simulink library "starslibAxisTransformations"  (R2024b)
settings: Solver=ode45  StartTime=0.0  StopTime=10.0  RelTol=1e-3  EnableMultiTasking=on
libraries: starslibMathOperations x25, $bdroot x18
(part 2 of 2)

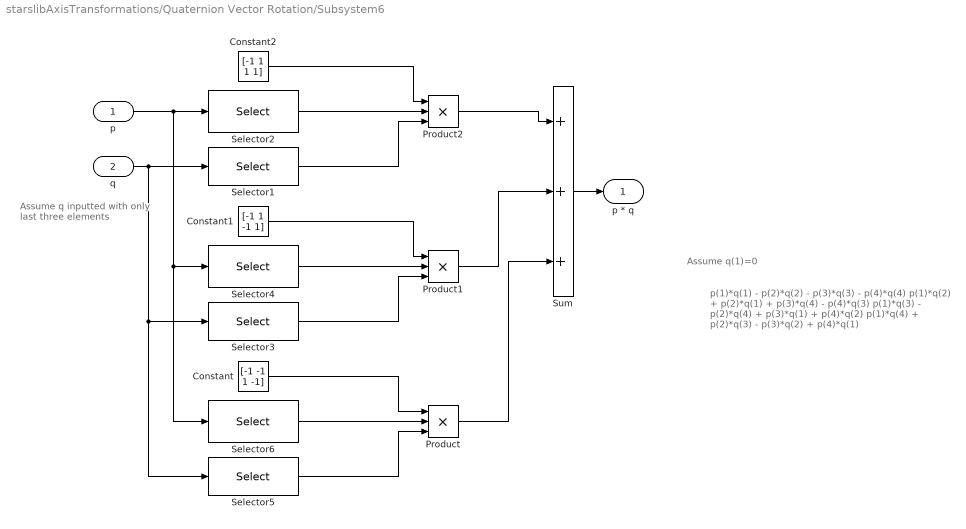
== system starslibAxisTransformations/Quaternion Vector Rotation/Subsystem6 ==
  note: p(1)*q(1) - p(2)*q(2) - p(3)*q(3) - p(4)*q(4)
      |
      | p(1)*q(2) + p(2)*q(1) + p(3)*q(4) - p(4)*q(3)
      |
      | p(1)*q(3) - p(2)*q(4) + p(3)*q(1) + p(4)*q(2)
      |
      | p(1)*q(4) + p(2)*q(3) - p(3)*q(2) + p(4)*q(1)
  note: Assume q(1)=0
  note: Assume q
      | inputted with only
      | last three elements
  p : Inport
  q : Inport  Port=2
  Constant : Constant  Value=[-1 -1 1 -1]
  Constant1 : Constant  Value=[-1 1 -1 1]
  Constant2 : Constant  Value=[-1 1 1 1]
  Product : Product  Inputs=3  RndMeth=Zero
  Product1 : Product  Inputs=3  RndMeth=Zero
  Product2 : Product  Inputs=3  RndMeth=Zero
  Selector1 : Selector  InputPortWidth=3  IndexOptions=Index vector (dialog)  Indices=[1 1 2 3]  OutputSizes=1
  Selector2 : Selector  InputPortWidth=4  IndexOptions=Index vector (dialog)  Indices=[2 1 1 1]  OutputSizes=1
  Selector3 : Selector  InputPortWidth=3  IndexOptions=Index vector (dialog)  Indices=[2 3 3 2]  OutputSizes=1
  Selector4 : Selector  InputPortWidth=4  IndexOptions=Index vector (dialog)  Indices=[3 3 2 2]  OutputSizes=1
  Selector5 : Selector  InputPortWidth=3  IndexOptions=Index vector (dialog)  Indices=[3 2 1 1]  OutputSizes=1
  Selector6 : Selector  InputPortWidth=4  IndexOptions=Index vector (dialog)  Indices=[4 4 4 3]  OutputSizes=1
  Sum : Sum  Inputs=+++
  p * q : Outport
  wires:
  Constant1/1 -> Product1/1
  Constant2/1 -> Product2/1
  Constant/1 -> Product/1
  Selector4/1 -> Product1/2
  Selector6/1 -> Product/2
  Selector1/1 -> Product2/3
  Selector3/1 -> Product1/3
  Selector5/1 -> Product/3
  Product2/1 -> Sum/1
  Product1/1 -> Sum/2
  Product/1 -> Sum/3
  p/1 -> Selector2/1, Selector4/1, Selector6/1
  q/1 -> Selector1/1, Selector3/1, Selector5/1
  Sum/1 -> p * q/1
  Selector2/1 -> Product2/2

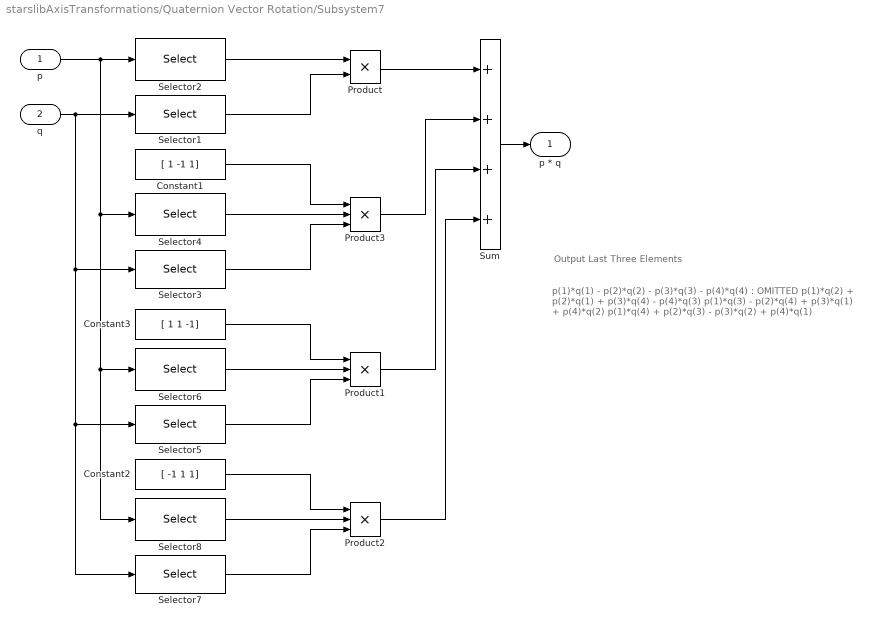
== system starslibAxisTransformations/Quaternion Vector Rotation/Subsystem7 ==
  note: Output Last Three Elements
  note: p(1)*q(1) - p(2)*q(2) - p(3)*q(3) - p(4)*q(4) :  OMITTED
      |
      | p(1)*q(2) + p(2)*q(1) + p(3)*q(4) - p(4)*q(3)
      |
      | p(1)*q(3) - p(2)*q(4) + p(3)*q(1) + p(4)*q(2)
      |
      | p(1)*q(4) + p(2)*q(3) - p(3)*q(2) + p(4)*q(1)
  p : Inport
  q : Inport  Port=2
  Constant1 : Constant  Value=[ 1 -1 1]
  Constant2 : Constant  Value=[ -1 1 1]
  Constant3 : Constant  Value=[ 1 1 -1]
  Product : Product  RndMeth=Zero
  Product1 : Product  Inputs=3  RndMeth=Zero
  Product2 : Product  Inputs=3  RndMeth=Zero
  Product3 : Product  Inputs=3  RndMeth=Zero
  Selector1 : Selector  InputPortWidth=4  IndexOptions=Index vector (dialog)  Indices=[ 2 3 4]  OutputSizes=1
  Selector2 : Selector  InputPortWidth=4  IndexOptions=Index vector (dialog)  Indices=[ 1 1 1]  OutputSizes=1
  Selector3 : Selector  InputPortWidth=4  IndexOptions=Index vector (dialog)  Indices=[ 1 4 3]  OutputSizes=1
  Selector4 : Selector  InputPortWidth=4  IndexOptions=Index vector (dialog)  Indices=[ 2 2 2]  OutputSizes=1
  Selector5 : Selector  InputPortWidth=4  IndexOptions=Index vector (dialog)  Indices=[ 4 1 2]  OutputSizes=1
  Selector6 : Selector  InputPortWidth=4  IndexOptions=Index vector (dialog)  Indices=[ 3 3 3]  OutputSizes=1
  Selector7 : Selector  InputPortWidth=4  IndexOptions=Index vector (dialog)  Indices=[ 3 2 1]  OutputSizes=1
  Selector8 : Selector  InputPortWidth=4  IndexOptions=Index vector (dialog)  Indices=[4 4 4]  OutputSizes=1
  Sum : Sum  Inputs=++++
  p * q : Outport
  wires:
  Selector5/1 -> Product1/3
  Selector6/1 -> Product1/2
  Constant3/1 -> Product1/1
  Selector7/1 -> Product2/3
  Selector8/1 -> Product2/2
  Constant2/1 -> Product2/1
  Selector3/1 -> Product3/3
  Selector4/1 -> Product3/2
  Constant1/1 -> Product3/1
  Selector1/1 -> Product/2
  Selector2/1 -> Product/1
  Sum/1 -> p * q/1
  q/1 -> Selector7/1, Selector5/1, Selector3/1, Selector1/1
  p/1 -> Selector8/1, Selector6/1, Selector4/1, Selector2/1
  Product2/1 -> Sum/4
  Product1/1 -> Sum/3
  Product3/1 -> Sum/2
  Product/1 -> Sum/1

== system starslibAxisTransformations/nQuaternion Decomposition/Divide by Zero Protection ==
  note: Replace magnitudes equal to 0 by 1
  M : Inport
  Constant : Constant
  Switch : Switch  Criteria=u2 ~= 0  ZeroCross=off  SaturateOnIntegerOverflow=off  InputSameDT=off
  M* : Outport
  wires:
  M/1 -> Switch/1, Switch/2
  Constant/1 -> Switch/3
  Switch/1 -> M*/1

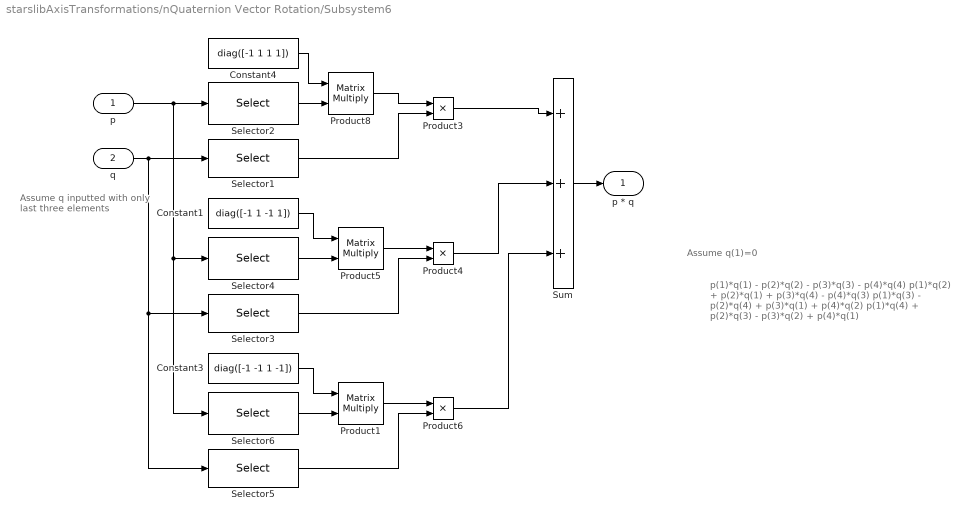
== system starslibAxisTransformations/nQuaternion Vector Rotation/Subsystem6 ==
  note: Assume q
      | inputted with only
      | last three elements
  note: Assume q(1)=0
  note: p(1)*q(1) - p(2)*q(2) - p(3)*q(3) - p(4)*q(4)
      |
      | p(1)*q(2) + p(2)*q(1) + p(3)*q(4) - p(4)*q(3)
      |
      | p(1)*q(3) - p(2)*q(4) + p(3)*q(1) + p(4)*q(2)
      |
      | p(1)*q(4) + p(2)*q(3) - p(3)*q(2) + p(4)*q(1)
  p : Inport  PortDimensions=[4,nQuat]
  q : Inport  Port=2  PortDimensions=[3,nQuat]
  Constant1 : Constant  Value=diag([-1 1 -1 1])  VectorParams1D=off
  Constant3 : Constant  Value=diag([-1 -1 1 -1])  VectorParams1D=off
  Constant4 : Constant  Value=diag([-1 1 1 1])  VectorParams1D=off
  Product1 : Product  Multiplication=Matrix(*)  RndMeth=Zero
  Product3 : Product  RndMeth=Zero
  Product4 : Product  RndMeth=Zero
  Product5 : Product  Multiplication=Matrix(*)  RndMeth=Zero
  Product6 : Product  RndMeth=Zero
  Product8 : Product  Multiplication=Matrix(*)  RndMeth=Zero
  Selector1 : Selector  NumberOfDimensions=2  InputPortWidth=3  IndexOptions=Index vector (dialog),Select all  Indices=[1 1 2 3],1  OutputSizes=1,1
  Selector2 : Selector  NumberOfDimensions=2  InputPortWidth=3  IndexOptions=Index vector (dialog),Select all  Indices=[2 1 1 1],1  OutputSizes=1,1
  Selector3 : Selector  NumberOfDimensions=2  InputPortWidth=3  IndexOptions=Index vector (dialog),Select all  Indices=[2 3 3 2],1  OutputSizes=1,1
  Selector4 : Selector  NumberOfDimensions=2  InputPortWidth=3  IndexOptions=Index vector (dialog),Select all  Indices=[3 3 2 2],1  OutputSizes=1,1
  Selector5 : Selector  NumberOfDimensions=2  InputPortWidth=3  IndexOptions=Index vector (dialog),Select all  Indices=[3 2 1 1],1  OutputSizes=1,1
  Selector6 : Selector  NumberOfDimensions=2  InputPortWidth=3  IndexOptions=Index vector (dialog),Select all  Indices=[4 4 4 3],1  OutputSizes=1,1
  Sum : Sum  Inputs=+++
  p * q : Outport  PortDimensions=[4,nQuat]
  wires:
  Constant4/1 -> Product8/1
  Product8/1 -> Product3/1
  Selector2/1 -> Product8/2
  Sum/1 -> p * q/1
  q/1 -> Selector5/1, Selector3/1, Selector1/1
  p/1 -> Selector6/1, Selector4/1, Selector2/1
  Product6/1 -> Sum/3
  Product4/1 -> Sum/2
  Product3/1 -> Sum/1
  Selector5/1 -> Product6/2
  Product1/1 -> Product6/1
  Selector3/1 -> Product4/2
  Product5/1 -> Product4/1
  Selector1/1 -> Product3/2
  Constant3/1 -> Product1/1
  Selector6/1 -> Product1/2
  Constant1/1 -> Product5/1
  Selector4/1 -> Product5/2

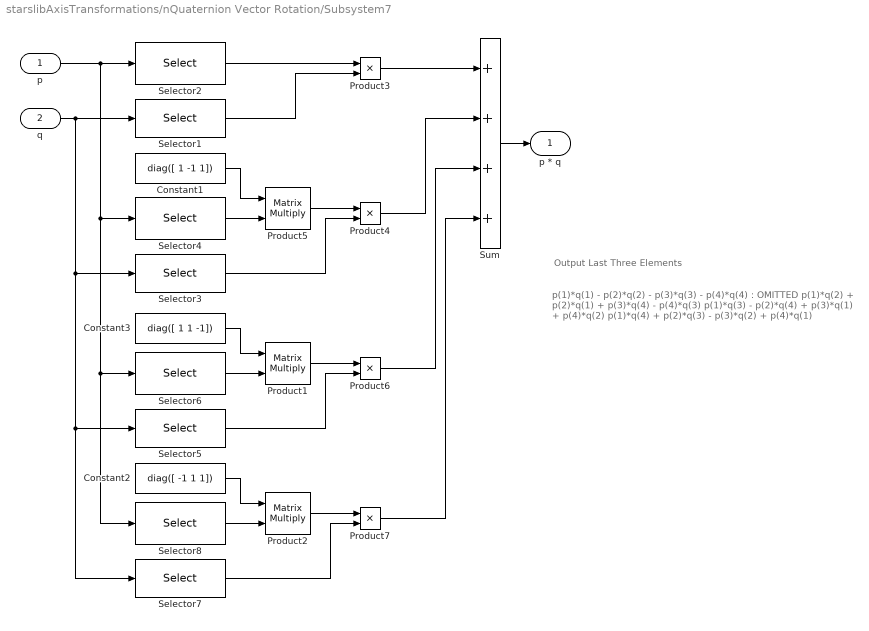
== system starslibAxisTransformations/nQuaternion Vector Rotation/Subsystem7 ==
  note: Output Last Three Elements
  note: p(1)*q(1) - p(2)*q(2) - p(3)*q(3) - p(4)*q(4) :  OMITTED
      |
      | p(1)*q(2) + p(2)*q(1) + p(3)*q(4) - p(4)*q(3)
      |
      | p(1)*q(3) - p(2)*q(4) + p(3)*q(1) + p(4)*q(2)
      |
      | p(1)*q(4) + p(2)*q(3) - p(3)*q(2) + p(4)*q(1)
  p : Inport  PortDimensions=[4,nQuat]
  q : Inport  Port=2  PortDimensions=[4,nQuat]
  Constant1 : Constant  Value=diag([ 1 -1 1])  VectorParams1D=off
  Constant2 : Constant  Value=diag([ -1 1 1])  VectorParams1D=off
  Constant3 : Constant  Value=diag([ 1 1 -1])  VectorParams1D=off
  Product1 : Product  Multiplication=Matrix(*)  RndMeth=Zero
  Product2 : Product  Multiplication=Matrix(*)  RndMeth=Zero
  Product{3..4,6..7} (4 alike) : Product  RndMeth=Zero
  Product5 : Product  Multiplication=Matrix(*)  RndMeth=Zero
  Selector1 : Selector  NumberOfDimensions=2  InputPortWidth=3  IndexOptions=Index vector (dialog),Select all  Indices=[ 2 3 4],1  OutputSizes=1,1
  Selector2 : Selector  NumberOfDimensions=2  InputPortWidth=3  IndexOptions=Index vector (dialog),Select all  Indices=[ 1 1 1],1  OutputSizes=1,1
  Selector3 : Selector  NumberOfDimensions=2  InputPortWidth=3  IndexOptions=Index vector (dialog),Select all  Indices=[ 1 4 3],1  OutputSizes=1,1
  Selector4 : Selector  NumberOfDimensions=2  InputPortWidth=3  IndexOptions=Index vector (dialog),Select all  Indices=[ 2 2 2],1  OutputSizes=1,1
  Selector5 : Selector  NumberOfDimensions=2  InputPortWidth=3  IndexOptions=Index vector (dialog),Select all  Indices=[ 4 1 2],1  OutputSizes=1,1
  Selector6 : Selector  NumberOfDimensions=2  InputPortWidth=3  IndexOptions=Index vector (dialog),Select all  Indices=[ 3 3 3],1  OutputSizes=1,1
  Selector7 : Selector  NumberOfDimensions=2  InputPortWidth=3  IndexOptions=Index vector (dialog),Select all  Indices=[ 3 2 1],1  OutputSizes=1,1
  Selector8 : Selector  NumberOfDimensions=2  InputPortWidth=3  IndexOptions=Index vector (dialog),Select all  Indices=[4 4 4],1  OutputSizes=1,1
  Sum : Sum  Inputs=++++
  p * q : Outport  PortDimensions=[3,nQuat]
  wires:
  Sum/1 -> p * q/1
  q/1 -> Selector7/1, Selector5/1, Selector3/1, Selector1/1
  p/1 -> Selector8/1, Selector6/1, Selector4/1, Selector2/1
  Product7/1 -> Sum/4
  Product6/1 -> Sum/3
  Product4/1 -> Sum/2
  Product3/1 -> Sum/1
  Selector7/1 -> Product7/2
  Product2/1 -> Product7/1
  Selector5/1 -> Product6/2
  Product1/1 -> Product6/1
  Selector3/1 -> Product4/2
  Product5/1 -> Product4/1
  Selector1/1 -> Product3/2
  Selector2/1 -> Product3/1
  Constant2/1 -> Product2/1
  Selector8/1 -> Product2/2
  Constant3/1 -> Product1/1
  Selector6/1 -> Product1/2
  Constant1/1 -> Product5/1
  Selector4/1 -> Product5/2

== system starslibAxisTransformations/slkQuaternion Vector Rotation/Subsystem6 ==
  note: Assume q
      | inputted with only
      | last three elements
  note: Assume q(1)=0
  note: p(1)*q(1) - p(2)*q(2) - p(3)*q(3) - p(4)*q(4)
      |
      | p(1)*q(2) + p(2)*q(1) + p(3)*q(4) - p(4)*q(3)
      |
      | p(1)*q(3) - p(2)*q(4) + p(3)*q(1) + p(4)*q(2)
      |
      | p(1)*q(4) + p(2)*q(3) - p(3)*q(2) + p(4)*q(1)
  p : Inport
  q : Inport  Port=2
  Constant : Constant  Value=[-1 -1 1 -1]
  Constant1 : Constant  Value=[-1 1 -1 1]
  Constant2 : Constant  Value=[-1 1 1 1]
  Product : Product  Inputs=3  RndMeth=Zero
  Product1 : Product  Inputs=3  RndMeth=Zero
  Product2 : Product  Inputs=3  RndMeth=Zero
  Selector1 : Selector  InputPortWidth=3  IndexOptions=Index vector (dialog)  Indices=[1 1 2 3]  OutputSizes=1
  Selector2 : Selector  InputPortWidth=4  IndexOptions=Index vector (dialog)  Indices=[2 1 1 1]  OutputSizes=1
  Selector3 : Selector  InputPortWidth=3  IndexOptions=Index vector (dialog)  Indices=[2 3 3 2]  OutputSizes=1
  Selector4 : Selector  InputPortWidth=4  IndexOptions=Index vector (dialog)  Indices=[3 3 2 2]  OutputSizes=1
  Selector5 : Selector  InputPortWidth=3  IndexOptions=Index vector (dialog)  Indices=[3 2 1 1]  OutputSizes=1
  Selector6 : Selector  InputPortWidth=4  IndexOptions=Index vector (dialog)  Indices=[4 4 4 3]  OutputSizes=1
  Sum : Sum  Inputs=+++
  p * q : Outport
  wires:
  Selector2/1 -> Product2/2
  Sum/1 -> p * q/1
  q/1 -> Selector5/1, Selector3/1, Selector1/1
  p/1 -> Selector6/1, Selector4/1, Selector2/1
  Product/1 -> Sum/3
  Product1/1 -> Sum/2
  Product2/1 -> Sum/1
  Selector5/1 -> Product/3
  Selector3/1 -> Product1/3
  Selector1/1 -> Product2/3
  Selector6/1 -> Product/2
  Selector4/1 -> Product1/2
  Constant/1 -> Product/1
  Constant2/1 -> Product2/1
  Constant1/1 -> Product1/1

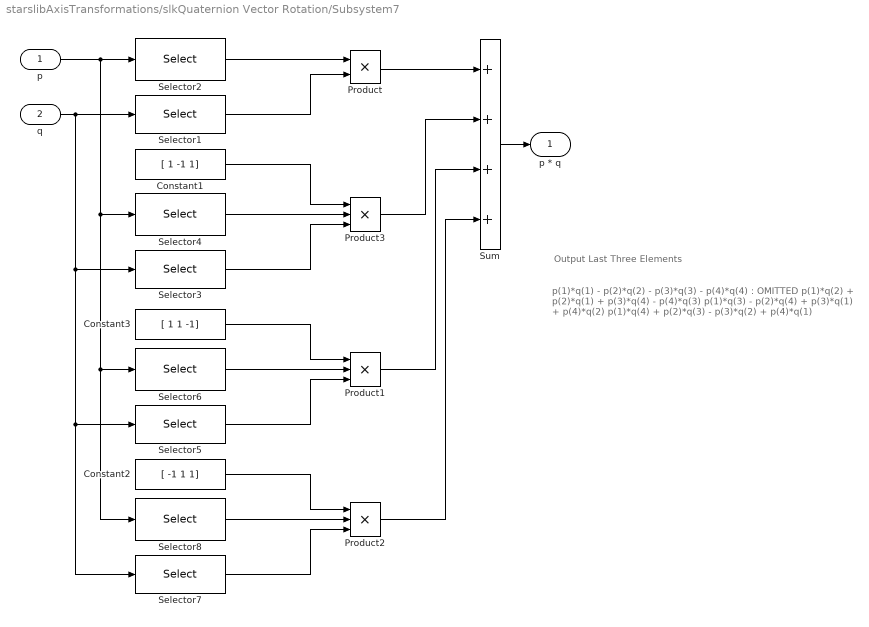
== system starslibAxisTransformations/slkQuaternion Vector Rotation/Subsystem7 ==
  note: p(1)*q(1) - p(2)*q(2) - p(3)*q(3) - p(4)*q(4) :  OMITTED
      |
      | p(1)*q(2) + p(2)*q(1) + p(3)*q(4) - p(4)*q(3)
      |
      | p(1)*q(3) - p(2)*q(4) + p(3)*q(1) + p(4)*q(2)
      |
      | p(1)*q(4) + p(2)*q(3) - p(3)*q(2) + p(4)*q(1)
  note: Output Last Three Elements
  p : Inport
  q : Inport  Port=2
  Constant1 : Constant  Value=[ 1 -1 1]
  Constant2 : Constant  Value=[ -1 1 1]
  Constant3 : Constant  Value=[ 1 1 -1]
  Product : Product  RndMeth=Zero
  Product1 : Product  Inputs=3  RndMeth=Zero
  Product2 : Product  Inputs=3  RndMeth=Zero
  Product3 : Product  Inputs=3  RndMeth=Zero
  Selector1 : Selector  InputPortWidth=4  IndexOptions=Index vector (dialog)  Indices=[ 2 3 4]  OutputSizes=1
  Selector2 : Selector  InputPortWidth=4  IndexOptions=Index vector (dialog)  Indices=[ 1 1 1]  OutputSizes=1
  Selector3 : Selector  InputPortWidth=4  IndexOptions=Index vector (dialog)  Indices=[ 1 4 3]  OutputSizes=1
  Selector4 : Selector  InputPortWidth=4  IndexOptions=Index vector (dialog)  Indices=[ 2 2 2]  OutputSizes=1
  Selector5 : Selector  InputPortWidth=4  IndexOptions=Index vector (dialog)  Indices=[ 4 1 2]  OutputSizes=1
  Selector6 : Selector  InputPortWidth=4  IndexOptions=Index vector (dialog)  Indices=[ 3 3 3]  OutputSizes=1
  Selector7 : Selector  InputPortWidth=4  IndexOptions=Index vector (dialog)  Indices=[ 3 2 1]  OutputSizes=1
  Selector8 : Selector  InputPortWidth=4  IndexOptions=Index vector (dialog)  Indices=[4 4 4]  OutputSizes=1
  Sum : Sum  Inputs=++++
  p * q : Outport
  wires:
  Product/1 -> Sum/1
  Product3/1 -> Sum/2
  Product1/1 -> Sum/3
  Product2/1 -> Sum/4
  p/1 -> Selector2/1, Selector4/1, Selector6/1, Selector8/1
  q/1 -> Selector1/1, Selector3/1, Selector5/1, Selector7/1
  Sum/1 -> p * q/1
  Selector2/1 -> Product/1
  Selector1/1 -> Product/2
  Constant1/1 -> Product3/1
  Selector4/1 -> Product3/2
  Selector3/1 -> Product3/3
  Constant2/1 -> Product2/1
  Selector8/1 -> Product2/2
  Selector7/1 -> Product2/3
  Constant3/1 -> Product1/1
  Selector6/1 -> Product1/2
  Selector5/1 -> Product1/3

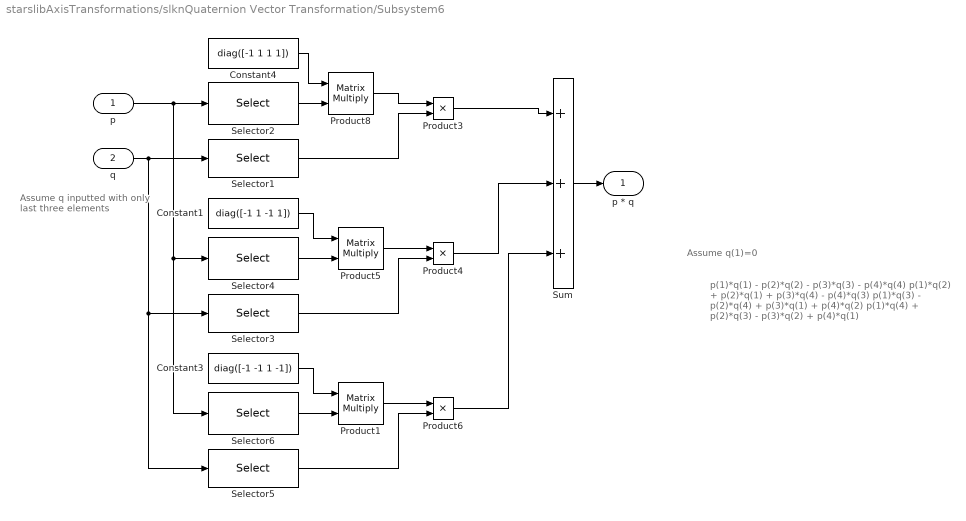
== system starslibAxisTransformations/slknQuaternion Vector Transformation/Subsystem6 ==
  note: Assume q
      | inputted with only
      | last three elements
  note: Assume q(1)=0
  note: p(1)*q(1) - p(2)*q(2) - p(3)*q(3) - p(4)*q(4)
      |
      | p(1)*q(2) + p(2)*q(1) + p(3)*q(4) - p(4)*q(3)
      |
      | p(1)*q(3) - p(2)*q(4) + p(3)*q(1) + p(4)*q(2)
      |
      | p(1)*q(4) + p(2)*q(3) - p(3)*q(2) + p(4)*q(1)
  p : Inport  PortDimensions=[4,nQuat]
  q : Inport  Port=2  PortDimensions=[3,nQuat]
  Constant1 : Constant  Value=diag([-1 1 -1 1])  VectorParams1D=off
  Constant3 : Constant  Value=diag([-1 -1 1 -1])  VectorParams1D=off
  Constant4 : Constant  Value=diag([-1 1 1 1])  VectorParams1D=off
  Product1 : Product  Multiplication=Matrix(*)  RndMeth=Zero
  Product3 : Product  RndMeth=Zero
  Product4 : Product  RndMeth=Zero
  Product5 : Product  Multiplication=Matrix(*)  RndMeth=Zero
  Product6 : Product  RndMeth=Zero
  Product8 : Product  Multiplication=Matrix(*)  RndMeth=Zero
  Selector1 : Selector  NumberOfDimensions=2  InputPortWidth=3  IndexOptions=Index vector (dialog),Select all  Indices=[1 1 2 3],1  OutputSizes=1,1
  Selector2 : Selector  NumberOfDimensions=2  InputPortWidth=3  IndexOptions=Index vector (dialog),Select all  Indices=[2 1 1 1],1  OutputSizes=1,1
  Selector3 : Selector  NumberOfDimensions=2  InputPortWidth=3  IndexOptions=Index vector (dialog),Select all  Indices=[2 3 3 2],1  OutputSizes=1,1
  Selector4 : Selector  NumberOfDimensions=2  InputPortWidth=3  IndexOptions=Index vector (dialog),Select all  Indices=[3 3 2 2],1  OutputSizes=1,1
  Selector5 : Selector  NumberOfDimensions=2  InputPortWidth=3  IndexOptions=Index vector (dialog),Select all  Indices=[3 2 1 1],1  OutputSizes=1,1
  Selector6 : Selector  NumberOfDimensions=2  InputPortWidth=3  IndexOptions=Index vector (dialog),Select all  Indices=[4 4 4 3],1  OutputSizes=1,1
  Sum : Sum  Inputs=+++
  p * q : Outport  PortDimensions=[4,nQuat]
  wires:
  Constant4/1 -> Product8/1
  Product8/1 -> Product3/1
  Selector2/1 -> Product8/2
  Sum/1 -> p * q/1
  q/1 -> Selector5/1, Selector3/1, Selector1/1
  p/1 -> Selector6/1, Selector4/1, Selector2/1
  Product6/1 -> Sum/3
  Product4/1 -> Sum/2
  Product3/1 -> Sum/1
  Selector5/1 -> Product6/2
  Product1/1 -> Product6/1
  Selector3/1 -> Product4/2
  Product5/1 -> Product4/1
  Selector1/1 -> Product3/2
  Constant3/1 -> Product1/1
  Selector6/1 -> Product1/2
  Constant1/1 -> Product5/1
  Selector4/1 -> Product5/2

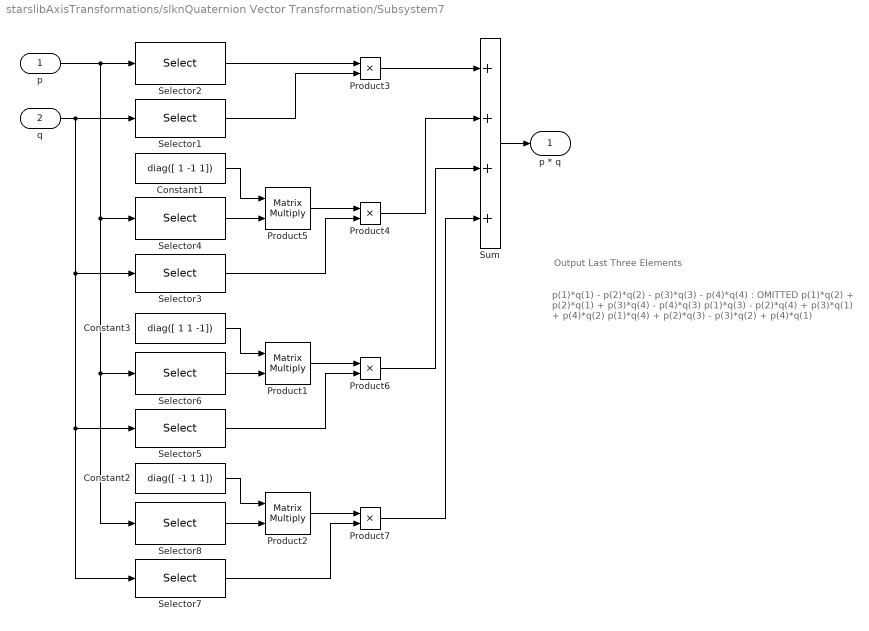
== system starslibAxisTransformations/slknQuaternion Vector Transformation/Subsystem7 ==
  note: Output Last Three Elements
  note: p(1)*q(1) - p(2)*q(2) - p(3)*q(3) - p(4)*q(4) :  OMITTED
      |
      | p(1)*q(2) + p(2)*q(1) + p(3)*q(4) - p(4)*q(3)
      |
      | p(1)*q(3) - p(2)*q(4) + p(3)*q(1) + p(4)*q(2)
      |
      | p(1)*q(4) + p(2)*q(3) - p(3)*q(2) + p(4)*q(1)
  p : Inport  PortDimensions=[4,nQuat]
  q : Inport  Port=2  PortDimensions=[4,nQuat]
  Constant1 : Constant  Value=diag([ 1 -1 1])  VectorParams1D=off
  Constant2 : Constant  Value=diag([ -1 1 1])  VectorParams1D=off
  Constant3 : Constant  Value=diag([ 1 1 -1])  VectorParams1D=off
  Product1 : Product  Multiplication=Matrix(*)  RndMeth=Zero
  Product2 : Product  Multiplication=Matrix(*)  RndMeth=Zero
  Product{3..4,6..7} (4 alike) : Product  RndMeth=Zero
  Product5 : Product  Multiplication=Matrix(*)  RndMeth=Zero
  Selector1 : Selector  NumberOfDimensions=2  InputPortWidth=3  IndexOptions=Index vector (dialog),Select all  Indices=[ 2 3 4],1  OutputSizes=1,1
  Selector2 : Selector  NumberOfDimensions=2  InputPortWidth=3  IndexOptions=Index vector (dialog),Select all  Indices=[ 1 1 1],1  OutputSizes=1,1
  Selector3 : Selector  NumberOfDimensions=2  InputPortWidth=3  IndexOptions=Index vector (dialog),Select all  Indices=[ 1 4 3],1  OutputSizes=1,1
  Selector4 : Selector  NumberOfDimensions=2  InputPortWidth=3  IndexOptions=Index vector (dialog),Select all  Indices=[ 2 2 2],1  OutputSizes=1,1
  Selector5 : Selector  NumberOfDimensions=2  InputPortWidth=3  IndexOptions=Index vector (dialog),Select all  Indices=[ 4 1 2],1  OutputSizes=1,1
  Selector6 : Selector  NumberOfDimensions=2  InputPortWidth=3  IndexOptions=Index vector (dialog),Select all  Indices=[ 3 3 3],1  OutputSizes=1,1
  Selector7 : Selector  NumberOfDimensions=2  InputPortWidth=3  IndexOptions=Index vector (dialog),Select all  Indices=[ 3 2 1],1  OutputSizes=1,1
  Selector8 : Selector  NumberOfDimensions=2  InputPortWidth=3  IndexOptions=Index vector (dialog),Select all  Indices=[4 4 4],1  OutputSizes=1,1
  Sum : Sum  Inputs=++++
  p * q : Outport  PortDimensions=[3,nQuat]
  wires:
  Sum/1 -> p * q/1
  q/1 -> Selector7/1, Selector5/1, Selector3/1, Selector1/1
  p/1 -> Selector8/1, Selector6/1, Selector4/1, Selector2/1
  Product7/1 -> Sum/4
  Product6/1 -> Sum/3
  Product4/1 -> Sum/2
  Product3/1 -> Sum/1
  Selector7/1 -> Product7/2
  Product2/1 -> Product7/1
  Selector5/1 -> Product6/2
  Product1/1 -> Product6/1
  Selector3/1 -> Product4/2
  Product5/1 -> Product4/1
  Selector1/1 -> Product3/2
  Selector2/1 -> Product3/1
  Constant2/1 -> Product2/1
  Selector8/1 -> Product2/2
  Constant3/1 -> Product1/1
  Selector6/1 -> Product1/2
  Constant1/1 -> Product5/1
  Selector4/1 -> Product5/2

== matlab function starslibAxisTransformations/funnQuaternion to Euler/Quaternion to Euler1 ==
  data: q input; rx output; n input; RotOrdVec input; ry output; rz output; U1 input; DirCrx input
function [rx, ry, rz] = fcn(q, n, RotOrdVec, U1, DirCrx )

[rx, ry, rz] = Quat2Euler(q, RotOrdVec,  U1, DirCrx);

% Ensure output vector dimensions 
rx = rx(n);
ry = ry(n);
rz = rz(n);

== matlab function starslibAxisTransformations/funQuaternion Vector Transformation/MATLAB Function ==
  data: q input; V_b output; V_a input
function V_b = QuaternionVectorTransformation(q, V_a) %#codegen
% Replaces the Simulink-block implementation of quaternion vector
% transformations so as to reduce block count. 

% For now (lazily), the existing function Qtrans is used, instead of 
% replicating the operations coded in the original block.  
% TODO: check that it works properly/does not consume excessive resources.
V_b = Qtrans(q,V_a);




end

== matlab function starslibAxisTransformations/funQuaternion to DCM/MATLAB Function ==
  data: q_in input; DCM output
function DCM = Quaternion2DCM(q_in)
% Directly reproduces Simulink block-based computation. 

[q,~,t] = qcheck4(q_in, 4);

var_1 = (q(1,1).^2 - sum(q(1,2:4).^2)) * eye(3);

var_2 = 2*(q(1,2:4)'*q(1,2:4)); %vector outer product

var_3 = ([0 1 -1; -1 0 1; 1 -1 0]'.*q([1 3 2; 3 2 1; 2 1 3]+1)) .*  q(1) * 2;

DCM = var_1 + var_2 - var_3;
